simulink model "DoPe"  (R2018a)
settings: Solver=VariableStepAuto  StartTime=0.0  StopTime=100  RelTol=1e-3
undefined symbols (not defined in the file): g, l1, l2, m1, m2
libraries: simulink x1
settings Model: Creator=Gerardo Berni  LastModifiedBy=Gerardo Berni
settings SolverCC: AlgebraicLoopSolver=LineSearch

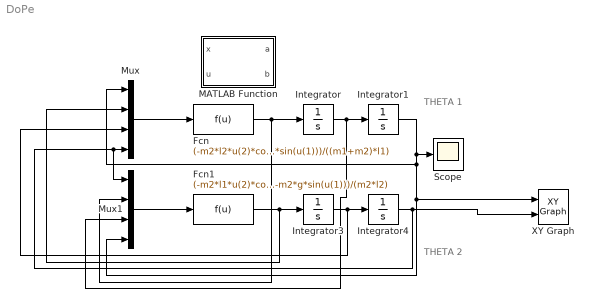
== system DoPe ==
  note: THETA 1
  note: THETA 2
  Fcn : Fcn  Expr=(-m2*l2*u(2)*cos(u(1)-u(4))-m2*l2*u(3)^2*sin(u(1)-u(4))-g*(m1+m2)*sin(u(1)))/((m1+m2)*l1)
  Fcn1 : Fcn  Expr=(-m2*l1*u(2)*cos(u(4)-u(1))+m2*l1*u(3)^2*sin(u(4)-u(1))-m2*g*sin(u(1)))/(m2*l2)
  Integrator : Integrator
  Integrator1 : Integrator  InitialCondition=pi/8
  Integrator3 : Integrator
  Integrator4 : Integrator
  MATLAB Function : MATLAB Function  TreatAsAtomicUnit=on
  Mux : Mux
  Mux1 : Mux
  Scope : Scope
  XY Graph : simulink/Sinks/XY Graph  xmin=-1  xmax=1  ymin=-1  ymax=1  st=-1
  wires:
  Integrator3/1 -> Mux/3, Integrator4/1
  Fcn/1 -> Mux1/2, Integrator/1
  Fcn1/1 -> Mux/2, Integrator3/1
  Mux/1 -> Fcn/1
  Mux1/1 -> Fcn1/1
  Integrator1/1 -> Mux1/4, XY Graph/1, Mux/1, Scope/1
  Integrator4/1 -> XY Graph/2, Mux1/1, Mux/4
  Integrator/1 -> Mux1/3, Integrator1/1

== matlab function DoPe/MATLAB Function ==
  data: x input; u input; a output; b output
function [a,b] = fcn(x,u)

a = x-u;
b = sin(x)-sqrt(u);
